simulink model "Test_simple_point_absorber"  (R2016b)
settings: Solver=VariableStepAuto  StartTime=0.0  StopTime=90.0  RelTol=1e-3
undefined symbols (not defined in the file or in its folder): seasetup
libraries: wave_simulations_library x1
settings Model: Creator=rcrozier  LastModifiedBy=rcrozier

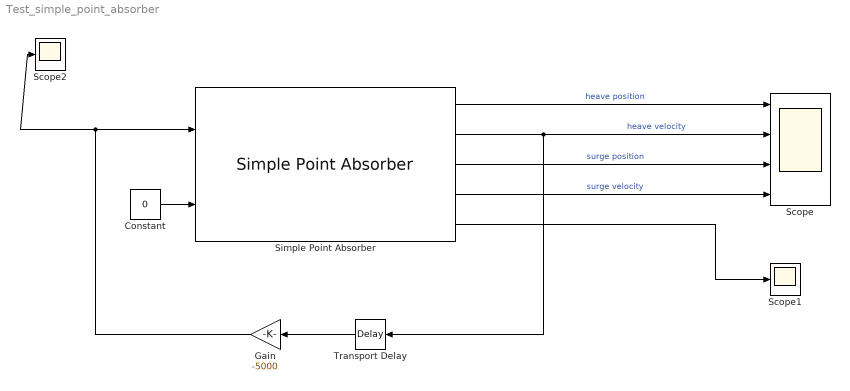
== system Test_simple_point_absorber ==
  Constant : Constant  Value=0
  Gain : Gain  Gain=-5000
  Scope : Scope  NumInputPorts=4
  Scope1 : Scope
  Scope2 : Scope
  Simple Point Absorber : wave_simulations_library/Simple Point Absorber  Buoy='cyl_2dia_1dr'  SeaParams=seasetup ('Sigmas', 2 * pi * 0.35)  NRadiationCoefs=10
  Transport Delay : TransportDelay  DelayTime=1e-6
  wires:
  Transport Delay/1 -> Gain/1
  Simple Point Absorber/2 -> Scope/2, Transport Delay/1  "heave velocity"
  Gain/1 -> Scope2/1, Simple Point Absorber/1
  Constant/1 -> Simple Point Absorber/2
  Simple Point Absorber/1 -> Scope/1  "heave position"
  Simple Point Absorber/3 -> Scope/3  "surge position"
  Simple Point Absorber/4 -> Scope/4  "surge velocity"
  Simple Point Absorber/5 -> Scope1/1
